simulink model "Fodiator_model"  (R2016a)
settings: Solver=VariableStepAuto  StartTime=0.0  StopTime=50  RelTol=1e-3
values from neighbouring files (symbols this model uses):
  alpha_AoA = [-12.75 -12.5 -12.25 -12 -11.75 -11.5 -11.25 -11 -10.75 -10.5 -10.25 -10 ... (297 elements, 99x3)]    [matlab.mat]
  Thrust_vs_PWM = [1100 1110 1120 1130 1140 1150 1160 1170 1180 1190 1200 1210 ... (243 elements, 81x3)]    [Thrust_PWM.mat]    (also in matlab.mat)
settings Model: Creator=abhij  LastModifiedBy=abhij

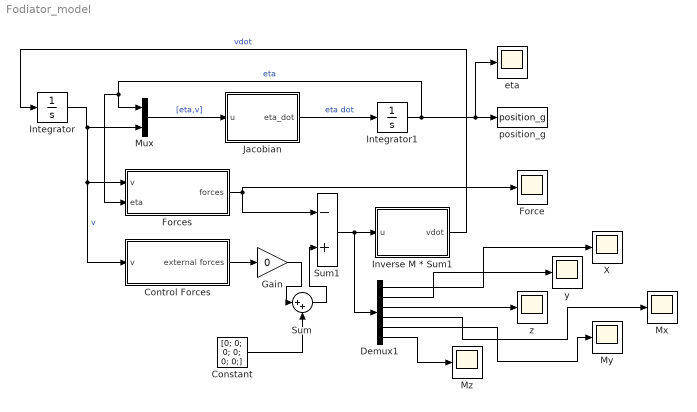
== system Fodiator_model ==
  Constant : Constant  Value=[0; 0; 0; 0; 0; 0;]
  Control Forces : Subsystem
  Demux1 : Demux  Outputs=6
  Force : Scope
  Forces : Subsystem
  Gain : Gain  Gain=0
  Integrator : Integrator  InitialCondition=[0;0;0;0;0;0]
  Integrator1 : Integrator  InitialCondition=[0;0;0;0;0;0]
  Inverse M * Sum1 : MATLAB Function  TreatAsAtomicUnit=on
  Jacobian : MATLAB Function  TreatAsAtomicUnit=on
  Mux : Mux  Inputs=2
  Mx : Scope
  My : Scope
  Mz : Scope
  Sum : Sum  Inputs=|++
  Sum1 : Sum  Inputs=-+
  X : Scope
  eta : Scope
  position_g : ToWorkspace  VariableName=position_g  SaveFormat=Timeseries  SampleTime=-1
  y : Scope
  "z " : Scope
  wires:
  Integrator/1 -> Control Forces/1(v), Forces/1(v), Mux/2  "v"
  Mux/1 -> Jacobian/1(u)  "[eta,v]"
  Jacobian/1(eta_dot) -> Integrator1/1  "eta dot"
  Integrator1/1 -> Forces/2(eta), Mux/1, eta/1, position_g/1  "eta"
  Sum1/1 -> Demux1/1, Inverse M * Sum1/1(u)
  Inverse M * Sum1/1(vdot) -> Integrator/1  "vdot"
  Forces/1(forces) -> Sum1/1, Force/1
  Control Forces/1(external forces) -> Gain/1
  Demux1/3 -> "z "/1
  Demux1/1 -> X/1
  Demux1/2 -> y/1
  Demux1/4 -> Mx/1
  Demux1/5 -> My/1
  Demux1/6 -> Mz/1
  Constant/1 -> Sum/2
  Gain/1 -> Sum/1
  Sum/1 -> Sum1/2

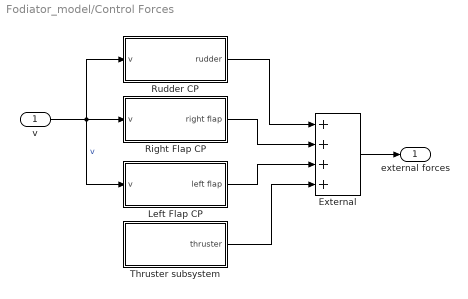
== system Fodiator_model/Control Forces ==
  v : Inport
  "External " : Sum  Inputs=++++
  Left Flap CP : Subsystem
  Right Flap CP : Subsystem
  Rudder CP : Subsystem
  Thruster subsystem : Subsystem
  external forces : Outport
  wires:
  v/1 -> Rudder CP/1(v), Left Flap CP/1(v), Right Flap CP/1(v)  "v"
  Rudder CP/1("rudder ") -> "External "/1
  "External "/1 -> external forces/1
  Right Flap CP/1(right flap) -> "External "/2
  Left Flap CP/1(left flap) -> "External "/3
  Thruster subsystem/1(thruster) -> "External "/4

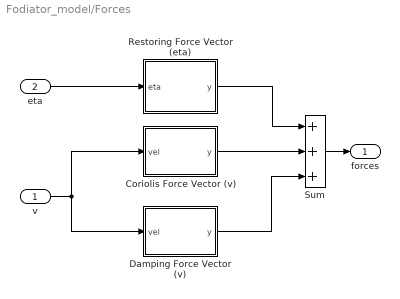
== system Fodiator_model/Forces ==
  v : Inport
  eta : Inport  Port=2
  Coriolis Force Vector (v) : MATLAB Function  TreatAsAtomicUnit=on
  Damping Force Vector (v) : MATLAB Function  TreatAsAtomicUnit=on
  Restoring Force Vector (eta) : MATLAB Function  TreatAsAtomicUnit=on
  Sum : Sum  Inputs=+++
  forces : Outport
  wires:
  Restoring Force Vector (eta)/1(y) -> Sum/1
  Coriolis Force Vector (v)/1(y) -> Sum/2
  Damping Force Vector (v)/1(y) -> Sum/3
  Sum/1 -> forces/1
  v/1 -> Coriolis Force Vector (v)/1(vel), Damping Force Vector (v)/1(vel)
  eta/1 -> Restoring Force Vector (eta)/1(eta)

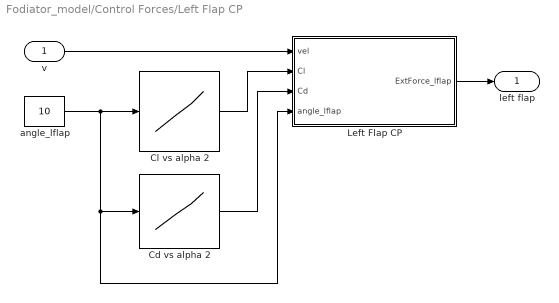
== system Fodiator_model/Control Forces/Left Flap CP ==
  v : Inport
  Cd vs alpha 2 : Lookup_n-D  NumberOfTableDimensions=1  BreakpointsForDimension1=alpha_AoA(:,1)  Table=alpha_AoA(:,2)  InternalRulePriority=Speed  RndMeth=Simplest  InputSameDT=on
  Cl vs alpha 2 : Lookup_n-D  NumberOfTableDimensions=1  BreakpointsForDimension1=alpha_AoA(:,1)  Table=alpha_AoA(:,3)  InternalRulePriority=Speed  RndMeth=Simplest  InputSameDT=on
  Left Flap CP : MATLAB Function  TreatAsAtomicUnit=on
  angle_lflap : Constant  Value=10
  left flap : Outport
  wires:
  v/1 -> Left Flap CP/1(vel)
  Left Flap CP/1(ExtForce_lflap) -> left flap/1
  angle_lflap/1 -> Left Flap CP/4(angle_lflap), Cd vs alpha 2/1, Cl vs alpha 2/1
  Cl vs alpha 2/1 -> Left Flap CP/2(Cl)
  Cd vs alpha 2/1 -> Left Flap CP/3(Cd)

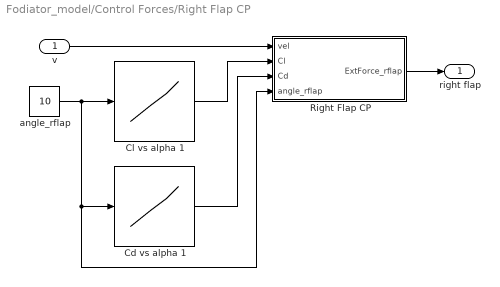
== system Fodiator_model/Control Forces/Right Flap CP ==
  v : Inport
  Cd vs alpha 1 : Lookup_n-D  NumberOfTableDimensions=1  BreakpointsForDimension1=alpha_AoA(:,1)  Table=alpha_AoA(:,2)  InternalRulePriority=Speed  RndMeth=Simplest  InputSameDT=on
  Cl vs alpha 1 : Lookup_n-D  NumberOfTableDimensions=1  BreakpointsForDimension1=alpha_AoA(:,1)  Table=alpha_AoA(:,3)  InternalRulePriority=Speed  RndMeth=Simplest  InputSameDT=on
  Right Flap CP : MATLAB Function  TreatAsAtomicUnit=on
  angle_rflap : Constant  Value=10
  right flap : Outport
  wires:
  v/1 -> Right Flap CP/1(vel)
  Right Flap CP/1(ExtForce_rflap) -> right flap/1
  Cl vs alpha 1/1 -> Right Flap CP/2(Cl)
  Cd vs alpha 1/1 -> Right Flap CP/3(Cd)
  angle_rflap/1 -> Cl vs alpha 1/1, Cd vs alpha 1/1, Right Flap CP/4(angle_rflap)

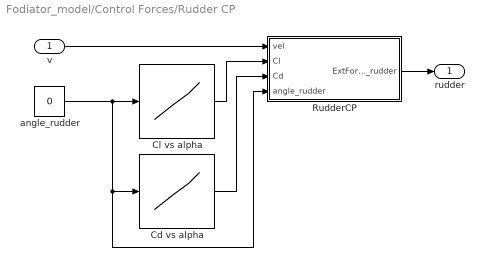
== system Fodiator_model/Control Forces/Rudder CP ==
  v : Inport
  "Cd vs alpha " : Lookup_n-D  NumberOfTableDimensions=1  BreakpointsForDimension1=alpha_AoA(:,1)  Table=alpha_AoA(:,2)  InternalRulePriority=Speed  RndMeth=Simplest  InputSameDT=on
  "Cl vs alpha " : Lookup_n-D  NumberOfTableDimensions=1  BreakpointsForDimension1=alpha_AoA(:,1)  Table=alpha_AoA(:,3)  InternalRulePriority=Speed  RndMeth=Simplest  InputSameDT=on
  "RudderCP " : MATLAB Function  TreatAsAtomicUnit=on
  angle_rudder : Constant  Value=0
  "rudder " : Outport
  wires:
  v/1 -> "RudderCP "/1(vel)
  "RudderCP "/1(ExtForce_rudder) -> "rudder "/1
  angle_rudder/1 -> "RudderCP "/4(angle_rudder), "Cd vs alpha "/1, "Cl vs alpha "/1
  "Cl vs alpha "/1 -> "RudderCP "/2(Cl)
  "Cd vs alpha "/1 -> "RudderCP "/3(Cd)

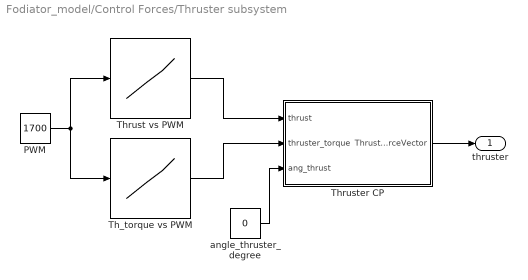
== system Fodiator_model/Control Forces/Thruster subsystem ==
  PWM : Constant  Value=1700
  Th_torque vs PWM : Lookup_n-D  NumberOfTableDimensions=1  BreakpointsForDimension1=Thrust_vs_PWM(:,1)  BreakpointsForDimension2=Thrust_vs_PWM(:,3)  Table=Thrust_vs_PWM(:,2)  InternalRulePriority=Speed  RndMeth=Simplest  InputSameDT=on
  Thrust vs PWM : Lookup_n-D  NumberOfTableDimensions=1  BreakpointsForDimension1=Thrust_vs_PWM(:,1)  BreakpointsForDimension2=Thrust_vs_PWM(:,3)  Table=Thrust_vs_PWM(:,2)  InternalRulePriority=Speed  RndMeth=Simplest  InputSameDT=on
  Thruster CP : MATLAB Function  TreatAsAtomicUnit=on
  angle_thruster_degree : Constant  Value=0
  thruster : Outport
  wires:
  Thruster CP/1(ThrusterForceVector) -> thruster/1
  PWM/1 -> Thrust vs PWM/1, Th_torque vs PWM/1
  angle_thruster_degree/1 -> Thruster CP/3(ang_thrust)
  Thrust vs PWM/1 -> Thruster CP/1(thrust)
  Th_torque vs PWM/1 -> Thruster CP/2(thruster_torque)

== matlab function Fodiator_model/Forces/Restoring Force Vector (eta) ==
  data: eta input; y output
function y = fcn(eta)
L=1.065;
R=0.125;
cb=[0 0 0]; %Centre of buyoancy
cg=[0 0 0]; %Centre of gravity
m=39;%mass of the vehicle
rho=1000;
b=8;

xg=cg(1);yg=cg(2);zg=cg(3);%Centre of gravity
xb=cb(1);yb=cb(2);zb=cb(3); % Centre of Buoyancy
W=m*9.81;B=(m+b)*9.81;

% Restoring efforts
G=[(W-B)*sin(eta(5));...
    -(W-B)*cos(eta(5))*sin(eta(4));...
    -(W-B)*cos(eta(5))*cos(eta(4));...
    -(yg*W-yb*B)*cos(eta(5))*cos(eta(4))+(zg*W-zb*B)*cos(eta(5))*sin(eta(4));...
  (zg*W-zb*B)*sin(eta(5))+(xg*W-xb*B)*cos(eta(5))*cos(eta(4));...
    -(xg*W-xb*B)*cos(eta(5))*sin(eta(4))-(yg*W-yb*B)*sin(eta(5))];
y=G;
end

== matlab function Fodiator_model/Jacobian ==
  data: u input; eta_dot output
function eta_dot = fcn(u)

v = u(7:12); %body_frame_velocities

phi=u(4); %roll
theta=u(5); %pitch
si=u(6);   %yaw
c_p=cos(phi);
c_t=cos(theta);
c_s=cos(si);
s_p=sin(phi);
s_t=sin(theta);
s_s=sin(si);
t_t=tan(theta);


J1=[c_s*c_t    -s_s*c_p+s_p*s_t*c_s     s_s*s_p+s_t*c_s*c_p;
    s_s*c_t     c_s*c_p+s_p*s_t*s_s    -c_s*s_p+s_t*s_s*c_p;
     -s_t            s_p*c_t                 c_p*c_t       ];
       
J2=[1      s_p*t_t     c_p*t_t;
    0        c_p        -s_p;
    0      s_p/c_t     c_p/c_t ];


J=[J1 zeros(3,3); zeros(3,3) J2];
eta_dot = J * v; % y == earth_velocities

end

== matlab function Fodiator_model/Forces/Coriolis Force Vector (v) ==
  data: vel input; y output
function y = Coriolis_Centripetal(vel) % Coriolis & Centripetal Matrix

L=1.065;
R=0.125;
cb=[0 0 0]; %Centre of buyoancy
cg=[0 0 0]; %Centre of gravity
m=39;%mass of the vehicle
rho=1000;

%Centre of gravity
xg=cg(1);yg=cg(2);zg=cg(3);%Centre of gravity

%Inertia values
ixy=0;iyx=ixy;ixz=0;izx=ixz;iyz=0;izy=iyz;
ix=0.34;iy=3.7;iz=3.7;

% Hydrodynamic derivatives
Xudot=-1.170; Xvdot=0; Xwdot=0; Xpdot=0; Xqdot=0; Xrdot=0;
Yudot=0; Yvdot=-34.834; Ywdot=0; Ypdot=0; Yqdot=0; Yrdot=1.042;
Zudot=0; Zvdot=0; Zwdot=-34.834; Zpdot=0; Zqdot=-1.042; Zrdot=0;
Kudot=0; Kvdot=0; Kwdot=0; Kpdot=0; Kqdot=0; Krdot=0;
Mudot=0; Mvdot=0; Mwdot=-1.042; Mpdot=0; Mqdot=-2.659; Mrdot=0; 
Nudot=0; Nvdot=-1.042; Nwdot=0; Npdot=0; Nqdot=0; Nrdot=-2.659;

% Coriolis and Centripetal Forces of Rigid body
Cvrb=[0 0 0 m*(yg*vel(5)+zg*vel(6)) -m*(xg*vel(5)-vel(3)) -m*(xg*vel(6)+vel(2));...
      0 0 0 -m*(yg*vel(4)+vel(3)) m*(zg*vel(6)+xg*vel(4)) -m*(yg*vel(6)-vel(1));...
      0 0 0 -m*(zg*vel(4)-vel(2)) -m*(zg*vel(5)+vel(1)) m*(xg*vel(4)+yg*vel(5));...
      -m*(yg*vel(5)+zg*vel(6)) m*(yg*vel(4)+vel(3)) m*(zg*vel(4)-vel(2)) 0 -iyz*vel(5)-ixz*vel(4)+iz*vel(6) iyz*vel(6)+ixy*vel(4)-iy*vel(5);...
      m*(xg*vel(5)-vel(3)) -m*(zg*vel(6)+xg*vel(4)) m*(zg*vel(5)+vel(1)) iyz*vel(5)+ixz*vel(4)-iz*vel(6) 0 -ixz*vel(6)-ixy*vel(5)+ix*vel(4);...
      m*(xg*vel(6)+vel(2)) m*(yg*vel(6)-vel(1)) -m*(xg*vel(4)+yg*vel(5)) -iyz*vel(6)-ixy*vel(4)+iy*vel(5) ixz*vel(6)+ixy*vel(5)-ix*vel(4) 0];

a1 = Xudot*vel(1)+Xvdot*vel(2)+Xwdot*vel(3)+Xpdot*vel(4)+Xqdot*vel(5)+Xrdot*vel(6);
a2 = Yudot*vel(1)+Yvdot*vel(2)+Ywdot*vel(3)+Ypdot*vel(4)+Yqdot*vel(5)+Yrdot*vel(6);
a3 = Zudot*vel(1)+Zvdot*vel(2)+Zwdot*vel(3)+Zpdot*vel(4)+Zqdot*vel(5)+Zrdot*vel(6);
b1 = Kudot*vel(1)+Kvdot*vel(2)+Kwdot*vel(3)+Kpdot*vel(4)+Kqdot*vel(5)+Krdot*vel(6);
b2 = Mudot*vel(1)+Mvdot*vel(2)+Mwdot*vel(3)+Mpdot*vel(4)+Mqdot*vel(5)+Mrdot*vel(6);
b3 = Nudot*vel(1)+Nvdot*vel(2)+Nwdot*vel(3)+Npdot*vel(4)+Nqdot*vel(5)+Nrdot*vel(6);
  
% Coriolis and Centripetal Forces of Added Mass
c1 = [0 -a3 a2;...
    a3 0 -a1;...
    -a2 a1 0];

c2 = [0 -b3 b2;...
    b3 0 -b1;...
    -b2 b1 0];

Ca=[zeros(3,3) c1;c1 c2];

C=Cvrb+Ca;
y=C*vel
end

== matlab function Fodiator_model/Forces/Damping Force Vector (v) ==
  data: vel input; y output

function y = Damping(vel) % Damping Matrix

L=1.065;
R=0.125;
cb=[0 0 0]; %Centre of buyoancy
cg=[0 0 0]; %Centre of gravity
m=39;%mass of the vehicle
rho=1000;

%velehicle Speed
U = sqrt(vel(1)^2+vel(2)^2+vel(3)^2);

%Hydrodynamic derivative details --to be modified for jubilee
Xu=-2.12; Xv=0; Xw=0; Xp=0; Xq=0; Xr=0;
Yu=0; Yv=-62.45; Yw=0; Yp=0; Yq=0; Yr=0.12;
Zu=0; Zv=0; Zw=-0.1749; Zp=0;  Zr=0;Zq=-0.066873;
Ku=0; Kv=0; Kw=0; Kp=0; Kq=0; Kr=0;
Mu=0; Mv=0;  Mp=0;  Mr=0;Mw=0;Mq=0;
Nu=0; Nv=1.2; Nw=0; Np=0; Nq=0; Nr=-31.25;
%jubilee parameters
Xuu=-7.365;Xvv=0;Xww=-0.737;Xpp=0;Xqq=-1.065;Xrr=-1.065;
Yuu=0;Yvv=-112.2;Yww=0;Ypp=0;Yqq=0;Yrr=0.250;
Zuu=0;Zvv=0;Zww=-112.2;Zpp=0;Zqq=-0.250;Zrr=0;
Kuu=0;Kvv=0;Kww=0;Kpp=0;Kqq=0;Krr=0;
Muu=0;Mvv=0;Mww=2.244;Mpp=0;Mqq=-119.5;Mrr=0;
Nuu=0;Nvv=-2.244;Nww=0;Npp=0;Nqq=0;Nrr=-59.75;

% Linear Damping Matrix
Dvl=-[Xu Xv Xw Xp Xq Xr;...
    Yu Yv Yw Yp Yq Yr;...
    Zu Zv Zw Zp Zq Zr;...
    Ku Kv Kw Kp Kq  Kr ;...
    Mu Mv Mw Mp  Mq  Mr ;...
    Nu Nv Nw Np  Nq  Nr ];

% Quadratic Damping Matrix
Dvq = -[Xuu Xvv Xww Xpp Xqq Xrr;...
    Yuu Yvv Yww Ypp Yqq Yrr;...
    Zuu Zvv Zww Zpp Zqq Zrr;...
    Kuu Kvv Kww Kpp Kqq Krr;...
    Muu Mvv Mww Mpp Mqq Mrr;...
    Nuu Nvv Nww Npp Nqq Nrr];

D = Dvl + Dvq;
y=D*vel;

== matlab function Fodiator_model/Inverse M * Sum1 ==
  data: u input; vdot output
function vdot = fcn(u)
sum1 = u;

M_rb=[1462  0      0     0       0        0;
      0     1462   0     0       0        -32.16;
      0     0      1462  0       32.16    0;
      0     0      0     498.63  0        0;
      0     0      32.16 0       1850.34  0;
      0     -32.16 0     0       0        2348.97];
  
M_a=[323.10 0       0       0       0       0;
     0      1049.21 0       0       0       -999.04;
     0      0       7040.36 0       -277.20 0;
     0      0       0       645.85  0       0;
     0      0       -277.20 0       7045.28 0;
     0      -996.04 0       0       0       8584.25];
 
M=M_rb+M_a; 
vdot = inv(M)*sum1;

end

== matlab function Fodiator_model/Control Forces/Rudder CP/RudderCP  ==
  data: vel input; ExtForce_rudder output; Cl input; Cd input; angle_rudder input
function ExtForce_rudder = fcn(vel,Cl,Cd,angle_rudder)

u = vel(1);
v = vel(2);
rho = 1000;

angle_rad = angle_rudder*pi/180;
u0 = u*cos(angle_rad)-v*sin(angle_rad);
v0 = u*sin(angle_rad)+v*cos(angle_rad);

alpha = atan2(v0,u0);
V = u0*cos(alpha)+v0*sin(alpha);

A_rudder = 0.02;
a = 100; b= 200; rx = 135; rz =60; ry = 0;

D = (1/2)*Cl*rho*A_rudder*abs(V)*V;
L = (1/2)*Cd*rho*A_rudder*abs(V)*V;
Fx = (D*cos(angle_rad)-L*sin(angle_rad));
Fy = -(D*sin(angle_rad)+L*cos(angle_rad));
Fz =  0;
Mx = -Fy*(rz+(a/2));
My =  Fx*(rz+(a/2));
Mz =  Fx*(b/2)*sin(angle_rad)+Fy*(rx+(a/2));

ExtForce_rudder = [Fx;Fy;Fz;Mx;My;Mz];

end

== matlab function Fodiator_model/Control Forces/Right Flap CP/Right Flap CP ==
  data: vel input; ExtForce_rflap output; Cl input; Cd input; angle_rflap input
function ExtForce_rflap = fcn(vel,Cl,Cd,angle_rflap)

u = vel(1);
w = vel(3);
rho = 1000;

angle_rad = angle_rflap*pi/180;
u0 = u*cos(angle_rad)-w*sin(angle_rad);
w0 = u*sin(angle_rad)+w*cos(angle_rad);

alpha = -atan2(w0,u0);
V = u0*cos(alpha)+w0*sin(alpha);

A_rflap = 0.015;
a = 100; b= 150; rx = 90; rz = 30; ry = 88;

D = (1/2)*Cl*rho*A_rflap*V*abs(V);
L = (1/2)*Cd*rho*A_rflap*V*abs(V);
Fx = -(D*cos(angle_rad)+L*sin(angle_rad));
Fy =  0;
Fz =  (D*sin(angle_rad)-L*cos(angle_rad));
Mx =  Fz*(ry+(a/2));
My =  Fx*(rz+(b/2)*sin(angle_rad))+Fz*(rx+(b/2)*cos(angle_rad));
Mz =  Fx*(ry+(a/2));

ExtForce_rflap = [Fx;Fy;Fz;Mx;My;Mz];

end

== matlab function Fodiator_model/Control Forces/Left Flap CP/Left Flap CP ==
  data: vel input; ExtForce_lflap output; Cl input; Cd input; angle_lflap input
function ExtForce_lflap = fcn(vel,Cl,Cd,angle_lflap)

u = vel(1);
w = vel(3);

angle_rad = angle_lflap*pi/180;
u0 = u*cos(angle_rad)-w*sin(angle_rad);
w0 = u*sin(angle_rad)+w*cos(angle_rad);

rho = 1000;

A_lflap = 0.015;
a = 100; b= 150; rx = 90; rz = 30; ry = 88;

alpha = -atan2(w0,u0);
V = u0*cos(alpha)+w0*sin(alpha);

D = (1/2)*Cl*rho*A_lflap*V*abs(V);
L = (1/2)*Cd*rho*A_lflap*V*abs(V);
Fx = -(D*cos(angle_rad)+L*sin(angle_rad));
Fy =  0;
Fz =  (D*sin(angle_rad)-L*cos(angle_rad));
Mx = -(Fz*(ry+(a/2)));
My =  Fx*(rz+(b/2)*sin(angle_rad))+Fz*(rx+(b/2)*cos(angle_rad));
Mz = -(Fx*(ry+(a/2)));

ExtForce_lflap = [Fx;Fy;Fz;Mx;My;Mz];

end

== matlab function Fodiator_model/Control Forces/Thruster subsystem/Thruster CP ==
  data: thrust input; thruster_torque input; ThrusterForceVector output; ang_thrust input
function ThrusterForceVector = fcn(thrust,thruster_torque,ang_thrust)

ang_rad_th = ang_thrust*(pi/180);
zth=0.07;
xth=0.02;
Mth=thruster_torque;

Fx = thrust*cos(ang_rad_th);
Fy = 0;
Fz = thrust*sin(ang_rad_th);
Mx = Mth*cos(ang_rad_th);
My = Fx*zth+Fz*xth;
Mz = Mth*sin(ang_rad_th); 


ThrusterForceVector = [Fx;Fy;Fz;Mx;My;Mz];

end
